simulink model "Mobile_robot_2wheels_PID_4_10_V0_2018 (1)"  (R2018b)
settings: Solver=VariableStepAuto  StartTime=0.0  StopTime=25  FixedStep=0.0001  MaxStep=0.01  RelTol=1e-3
libraries: fuzblock x6, simulink x4
settings Model: Creator=HP-PC  LastModifiedBy=thetr
settings DebuggingCC: SFMachineParentedDataDiag=error

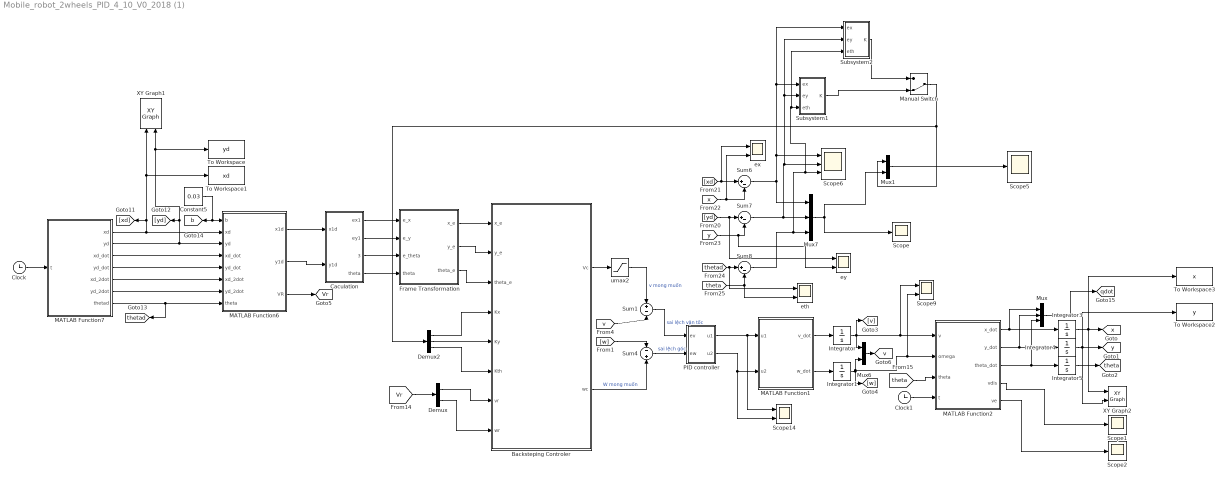
== system Mobile_robot_2wheels_PID_4_10_V0_2018 (1) ==
  Backsteping Controler : MATLAB Function  TreatAsAtomicUnit=on
  Caculation : Subsystem
  Clock : Clock
  Clock1 : Clock
  Constant5 : Constant  Value=0.03
  Demux : Demux  Outputs=2
  Demux2 : Demux  Outputs=3
  Frame Transformation : MATLAB Function  TreatAsAtomicUnit=on
  Integrator{,1,3..5} (5 alike) : Integrator
  MATLAB Function1 : MATLAB Function  TreatAsAtomicUnit=on
  MATLAB Function2 : MATLAB Function  TreatAsAtomicUnit=on
  MATLAB Function6 : MATLAB Function  TreatAsAtomicUnit=on
  MATLAB Function7 : MATLAB Function  TreatAsAtomicUnit=on
  Manual Switch : ManualSwitch  CurrentSetting=0
  Mux : Mux  Inputs=3
  Mux1 : Mux  Inputs=2
  Mux6 : Mux  Inputs=2
  Mux7 : Mux  Inputs=3
  PID controller : Subsystem
  Scope{,1..2,5} (4 alike) : Scope
  Scope14 : Scope  NumInputPorts=2
  Scope6 : Scope  NumInputPorts=3
  Scope9 : Scope  NumInputPorts=2
  Subsystem1 : Subsystem
  Subsystem2 : Subsystem
  Sum1 : Sum  Inputs=+-
  Sum4 : Sum  Inputs=-+
  Sum6 : Sum  Inputs=|+-
  Sum7 : Sum  Inputs=|+-
  Sum8 : Sum  Inputs=|+-
  To Workspace : ToWorkspace  VariableName=yd  SampleTime=-1
  To Workspace1 : ToWorkspace  VariableName=xd  SampleTime=-1
  To Workspace2 : ToWorkspace  VariableName=y  SampleTime=-1
  To Workspace3 : ToWorkspace  VariableName=x  SampleTime=-1
  XY Graph1 : simulink/Sinks/XY Graph  xmin=-20  xmax=20  ymin=-20  ymax=20  st=-1
  XY Graph2 : simulink/Sinks/XY Graph  xmin=-20  xmax=20  ymin=-20  ymax=20  st=-1
  eth : Scope  NumInputPorts=2
  ex : Scope  NumInputPorts=2
  ey : Scope  NumInputPorts=2
  umax2 : Saturate  UpperLimit=3  LowerLimit=-3
  tag scope: Vr=global, b=global, qdot=global, theta=global, thetad=global, v=global, x=global, y=global
  wires:
  Integrator4/1 -> To Workspace2/1, XY Graph2/2, [y]
  Integrator5/1 -> [theta]
  Integrator3/1 -> To Workspace3/1, XY Graph2/1, [x]
  MATLAB Function7/1(xd) -> To Workspace1/1, XY Graph1/1, [xd], MATLAB Function6/2(xd)
  MATLAB Function2/3(theta_dot) -> Mux/3, Integrator5/1
  MATLAB Function2/1(x_dot) -> Integrator3/1, Mux/1
  PID controller/2(u2) -> Scope14/2, MATLAB Function1/2(u2)
  Demux2/2 -> Backsteping Controler/5(Ky)
  Frame Transformation/3(theta_e) -> Backsteping Controler/3(theta_e)
  PID controller/1(u1) -> Scope14/1, MATLAB Function1/1(u1)
  MATLAB Function1/2(w_dot) -> Integrator1/1
  Clock/1 -> MATLAB Function7/1(t)
  Constant5/1 -> MATLAB Function6/1(b), [b]
  MATLAB Function7/3(xd_dot) -> MATLAB Function6/4(xd_dot)
  MATLAB Function7/7(thetad) -> [thetad], MATLAB Function6/8(theta)
  Mux7/1 -> Scope/1, Mux1/2
  Sum1/1 -> PID controller/1(ev)  "sai lệch vận tốc"
  [x] -> ex/2, Sum6/2
  MATLAB Function7/2(yd) -> To Workspace/1, XY Graph1/2, [yd], MATLAB Function6/3(yd)
  Sum8/1 -> Subsystem2/3(eth), Subsystem1/3(eth), Scope6/3, Mux7/3
  [Vr] -> Demux/1
  [thetad] -> eth/1, Sum8/1
  Integrator1/1 -> Mux6/2, Scope9/2, MATLAB Function2/2(omega), [w]
  [xd] -> ex/1, Sum6/1
  Sum4/1 -> PID controller/2(ew)  "sai lệch góc"
  Frame Transformation/2(y_e) -> Backsteping Controler/2(y_e)
  Demux2/1 -> Backsteping Controler/4(Kx)
  [v] -> Sum1/2
  Caculation/4(theta) -> Frame Transformation/4(theta)
  Demux/2 -> Backsteping Controler/8(wr)
  [w] -> Sum4/1
  MATLAB Function1/1(v_dot) -> Integrator/1
  MATLAB Function6/1(x1d) -> Caculation/1(x1d)
  Caculation/1(ex1) -> Frame Transformation/1(e_x)
  MATLAB Function7/4(yd_dot) -> MATLAB Function6/5(yd_dot)
  Demux2/3 -> Backsteping Controler/6(Kth)
  Mux/1 -> [qdot]
  Demux/1 -> Backsteping Controler/7(vr)
  MATLAB Function6/3(VR) -> [Vr]
  [theta] -> eth/2, Sum8/2
  Clock1/1 -> MATLAB Function2/4(t)
  Frame Transformation/1(x_e) -> Backsteping Controler/1(x_e)
  umax2/1 -> Sum1/1  "v mong muốn"
  Integrator/1 -> [v], Scope9/1, MATLAB Function2/1(v), Mux6/1
  MATLAB Function7/5(xd_2dot) -> MATLAB Function6/6(xd_2dot)
  MATLAB Function7/6(yd_2dot) -> MATLAB Function6/7(yd_2dot)
  [theta] -> MATLAB Function2/3(theta)
  Caculation/3(etheta1) -> Frame Transformation/3(e_theta)
  MATLAB Function6/2(y1d) -> Caculation/2(y1d)
  MATLAB Function2/2(y_dot) -> Mux/2, Integrator4/1
  Caculation/2(ey1) -> Frame Transformation/2(e_y)
  Sum6/1 -> Subsystem2/1(ex), Subsystem1/1(ex), Scope6/1, Mux7/1
  Mux6/1 -> [v]
  [yd] -> ey/1, Sum7/1
  Backsteping Controler/1(Vc) -> umax2/1
  Sum7/1 -> Scope6/2, Subsystem2/2(ey), Subsystem1/2(ey), Mux7/2
  Backsteping Controler/2(wc) -> Sum4/2  "W mong muốn"
  Subsystem1/1(K) -> Manual Switch/2
  Mux1/1 -> Scope5/1
  MATLAB Function2/4(vdis) -> Scope1/1
  MATLAB Function2/5(ve) -> Scope2/1
  [y] -> ey/2, Sum7/2
  Subsystem2/1(K) -> Manual Switch/1
  Manual Switch/1 -> Demux2/1, Mux1/1

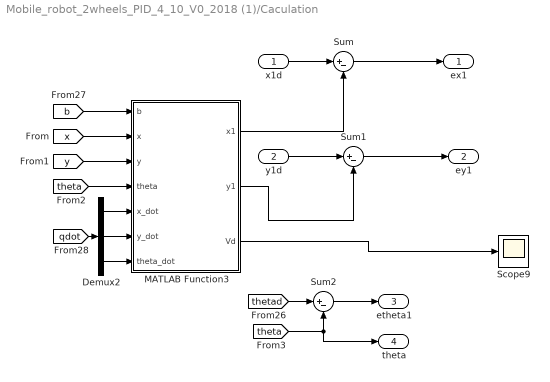
== system Mobile_robot_2wheels_PID_4_10_V0_2018 (1)/Caculation ==
  x1d : Inport
  y1d : Inport  Port=2
  Demux2 : Demux  Outputs=3
  MATLAB Function3 : MATLAB Function  TreatAsAtomicUnit=on
  Scope9 : Scope
  Sum : Sum  Inputs=|+-
  Sum1 : Sum  Inputs=|+-
  Sum2 : Sum  Inputs=|+-
  ex1 : Outport  VectorParamsAs1DForOutWhenUnconnected=on
  ey1 : Outport  Port=2  VectorParamsAs1DForOutWhenUnconnected=on
  etheta1 : Outport  Port=3  VectorParamsAs1DForOutWhenUnconnected=on
  theta : Outport  Port=4  VectorParamsAs1DForOutWhenUnconnected=on
  wires:
  Demux2/3 -> MATLAB Function3/7(theta_dot)
  MATLAB Function3/3(Vd) -> Scope9/1
  [y] -> MATLAB Function3/3(y)
  Sum/1 -> ex1/1
  MATLAB Function3/2(y1) -> Sum1/2
  MATLAB Function3/1(x1) -> Sum/2
  [x] -> MATLAB Function3/2(x)
  Demux2/2 -> MATLAB Function3/6(y_dot)
  [theta] -> MATLAB Function3/4(theta)
  [b] -> MATLAB Function3/1(b)
  Demux2/1 -> MATLAB Function3/5(x_dot)
  [qdot] -> Demux2/1
  Sum1/1 -> ey1/1
  y1d/1 -> Sum1/1
  x1d/1 -> Sum/1
  [thetad] -> Sum2/1
  [theta] -> theta/1, Sum2/2
  Sum2/1 -> etheta1/1

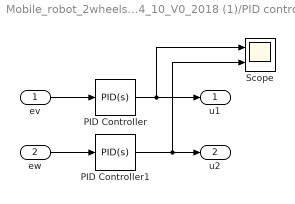
== system Mobile_robot_2wheels_PID_4_10_V0_2018 (1)/PID controller ==
  ev : Inport
  ew : Inport  Port=2
  PID Controller : simulink/Continuous/PID Controller  Controller=PID  Form=Parallel  TimeDomain=Continuous-time  SampleTime=-1  IntegratorMethod=Forward Euler  FilterMethod=Forward Euler  ControllerParametersSource=internal  P=100  I=10  D=0.1  UseFilter=on  N=193.352804132204  TunerSelectOption=Transfer Function Based (PID Tuner App)  InitialConditionSource=internal  InitialConditionForIntegrator=0  InitialConditionForFilter=0  DifferentiatorICPrevScaledInput=0  ExternalReset=none  TrackingMode=off  Kt=1  LimitOutput=off  UpperSaturationLimit=inf  LowerSaturationLimit=-inf  LinearizeAsGain=on  AntiWindupMode=none  Kb=1  POutMin=[]  POutMax=[]  IOutMin=[]  IOutMax=[]  DOutMin=[]  DOutMax=[]  NOutMin=[]  NOutMax=[]  SumOutMin=[]  SumOutMax=[]  SaturationOutMin=[]  SaturationOutMax=[]  PParamMin=[]  PParamMax=[]  IParamMin=[]  IParamMax=[]  DParamMin=[]  DParamMax=[]  NParamMin=[]  NParamMax=[]  KbParamMin=[]  KbParamMax=[]  KtParamMin=[]  KtParamMax=[]  KbOutMin=[]  KbOutMax=[]  KtOutMin=[]  KtOutMax=[]  IntegratorOutMin=[]  IntegratorOutMax=[]  FilterOutMin=[]  FilterOutMax=[]  SumI1OutMin=[]  SumI1OutMax=[]  SumI2OutMin=[]  SumI2OutMax=[]  SumI3OutMin=[]  SumI3OutMax=[]  SumI4OutMin=[]  SumI4OutMax=[]  SumDOutMin=[]  SumDOutMax=[]  DifferentiatorOutMin=[]  DifferentiatorOutMax=[]  FilterDiffOutCoefMin=[]  FilterDiffOutCoefMax=[]  ReciprocalOutMin=[]  ReciprocalOutMax=[]  SumDenOutMin=[]  SumDenOutMax=[]  SumNumOutMin=[]  SumNumOutMax=[]  DivideOutMin=[]  DivideOutMax=[]  IntegratorContinuousStateAttributes=''  IntegratorStateMustResolveToSignalObject=off  IntegratorRTWStateStorageClass=Auto  FilterContinuousStateAttributes=''  FilterStateMustResolveToSignalObject=off  FilterRTWStateStorageClass=Auto  ParallelPVariant=InternalParameters  IdealPVariant=Disabled  IVariant=InternalParameters  DVariant=InternalParameters  IntegratorVariant=Continuous  SatVariant=Disabled  AWVariant=Passthrough  PCopyVariant=Disabled  TRVariant=Disabled  FdbkBlocksVariant=Forward  IdealPFdbkVariant=Disabled  SatFdbkVariant=Disabled  DerivativeFilterVariant=ContFilter  NVariant=InternalParameters  NCopyVariant=Disabled  FilterICVariant=InternalICsFilter  IntegratorICVariant=InternalICs  ExternalResetVariant=Disabled  TRSumVariant=Passthrough  SumFdbkVariant=Disabled  SumVariant=Sum_PID
  PID Controller1 : simulink/Continuous/PID Controller  Controller=PID  Form=Parallel  TimeDomain=Continuous-time  SampleTime=-1  IntegratorMethod=Forward Euler  FilterMethod=Forward Euler  ControllerParametersSource=internal  P=100  I=10  D=0.1  UseFilter=on  N=3867.05608255163  TunerSelectOption=Transfer Function Based (PID Tuner App)  InitialConditionSource=internal  InitialConditionForIntegrator=0  InitialConditionForFilter=0  DifferentiatorICPrevScaledInput=0  ExternalReset=none  TrackingMode=off  Kt=1  LimitOutput=off  UpperSaturationLimit=inf  LowerSaturationLimit=-inf  LinearizeAsGain=on  AntiWindupMode=none  Kb=1  POutMin=[]  POutMax=[]  IOutMin=[]  IOutMax=[]  DOutMin=[]  DOutMax=[]  NOutMin=[]  NOutMax=[]  SumOutMin=[]  SumOutMax=[]  SaturationOutMin=[]  SaturationOutMax=[]  PParamMin=[]  PParamMax=[]  IParamMin=[]  IParamMax=[]  DParamMin=[]  DParamMax=[]  NParamMin=[]  NParamMax=[]  KbParamMin=[]  KbParamMax=[]  KtParamMin=[]  KtParamMax=[]  KbOutMin=[]  KbOutMax=[]  KtOutMin=[]  KtOutMax=[]  IntegratorOutMin=[]  IntegratorOutMax=[]  FilterOutMin=[]  FilterOutMax=[]  SumI1OutMin=[]  SumI1OutMax=[]  SumI2OutMin=[]  SumI2OutMax=[]  SumI3OutMin=[]  SumI3OutMax=[]  SumI4OutMin=[]  SumI4OutMax=[]  SumDOutMin=[]  SumDOutMax=[]  DifferentiatorOutMin=[]  DifferentiatorOutMax=[]  FilterDiffOutCoefMin=[]  FilterDiffOutCoefMax=[]  ReciprocalOutMin=[]  ReciprocalOutMax=[]  SumDenOutMin=[]  SumDenOutMax=[]  SumNumOutMin=[]  SumNumOutMax=[]  DivideOutMin=[]  DivideOutMax=[]  IntegratorContinuousStateAttributes=''  IntegratorStateMustResolveToSignalObject=off  IntegratorRTWStateStorageClass=Auto  FilterContinuousStateAttributes=''  FilterStateMustResolveToSignalObject=off  FilterRTWStateStorageClass=Auto  ParallelPVariant=InternalParameters  IdealPVariant=Disabled  IVariant=InternalParameters  DVariant=InternalParameters  IntegratorVariant=Continuous  SatVariant=Disabled  AWVariant=Passthrough  PCopyVariant=Disabled  TRVariant=Disabled  FdbkBlocksVariant=Forward  IdealPFdbkVariant=Disabled  SatFdbkVariant=Disabled  DerivativeFilterVariant=ContFilter  NVariant=InternalParameters  NCopyVariant=Disabled  FilterICVariant=InternalICsFilter  IntegratorICVariant=InternalICs  ExternalResetVariant=Disabled  TRSumVariant=Passthrough  SumFdbkVariant=Disabled  SumVariant=Sum_PID
  Scope : Scope  NumInputPorts=2
  u1 : Outport
  u2 : Outport  Port=2
  wires:
  ev/1 -> PID Controller/1
  ew/1 -> PID Controller1/1
  PID Controller/1 -> Scope/1, u1/1
  PID Controller1/1 -> Scope/2, u2/1

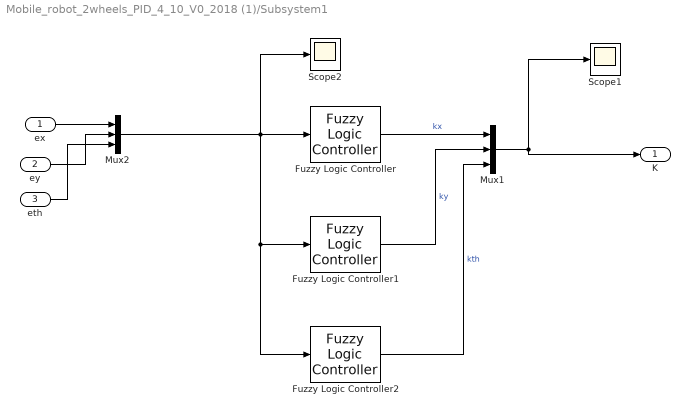
== system Mobile_robot_2wheels_PID_4_10_V0_2018 (1)/Subsystem1 ==
  ex : Inport
  ey : Inport  Port=2
  eth : Inport  Port=3
  Fuzzy Logic Controller : fuzblock/Fuzzy Logic  Controller  FIS='FUZZY1_1.fis'  OutputSampleNumber=101  DataType=double  FuzzifiedInputs=off  RuleFiringStrengths=off  RuleOutputs=off  AggregatedOutputs=off  SimulateUsing=Interpreted execution  OutOfRangeInputValueMessage=warning  NoRuleFiredMessage=warning  EmptyOutputFuzzySetMessage=warning
  Fuzzy Logic Controller1 : fuzblock/Fuzzy Logic  Controller  FIS='FUZZY1_2.fis'  OutputSampleNumber=101  DataType=double  FuzzifiedInputs=off  RuleFiringStrengths=off  RuleOutputs=off  AggregatedOutputs=off  SimulateUsing=Interpreted execution  OutOfRangeInputValueMessage=warning  NoRuleFiredMessage=warning  EmptyOutputFuzzySetMessage=warning
  Fuzzy Logic Controller2 : fuzblock/Fuzzy Logic  Controller  FIS='FUZZY1_3.fis'  OutputSampleNumber=101  DataType=double  FuzzifiedInputs=off  RuleFiringStrengths=off  RuleOutputs=off  AggregatedOutputs=off  SimulateUsing=Interpreted execution  OutOfRangeInputValueMessage=warning  NoRuleFiredMessage=warning  EmptyOutputFuzzySetMessage=warning
  Mux1 : Mux  Inputs=3
  Mux2 : Mux  Inputs=3
  Scope1 : Scope
  Scope2 : Scope
  K : Outport  VectorParamsAs1DForOutWhenUnconnected=on
  wires:
  Fuzzy Logic Controller/1 -> Mux1/1  "kx"
  Fuzzy Logic Controller2/1 -> Mux1/3  "kth"
  Fuzzy Logic Controller1/1 -> Mux1/2  "ky"
  Mux1/1 -> K/1, Scope1/1
  ex/1 -> Mux2/1
  Mux2/1 -> Fuzzy Logic Controller2/1, Fuzzy Logic Controller1/1, Scope2/1, Fuzzy Logic Controller/1
  ey/1 -> Mux2/2
  eth/1 -> Mux2/3

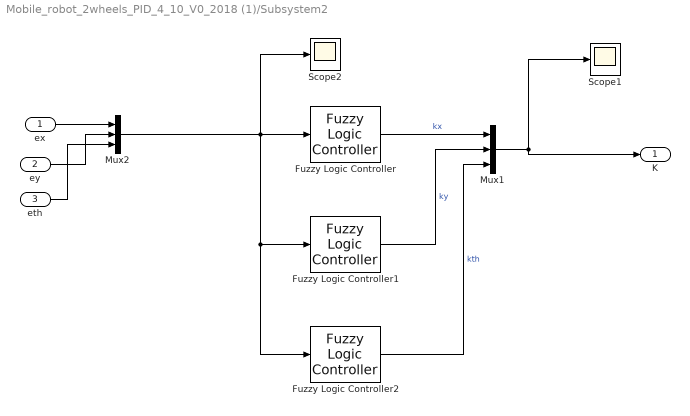
== system Mobile_robot_2wheels_PID_4_10_V0_2018 (1)/Subsystem2 ==
  ex : Inport
  ey : Inport  Port=2
  eth : Inport  Port=3
  Fuzzy Logic Controller : fuzblock/Fuzzy Logic  Controller  FIS='LUAT9B1.fis'  OutputSampleNumber=101  DataType=double  FuzzifiedInputs=off  RuleFiringStrengths=off  RuleOutputs=off  AggregatedOutputs=off  SimulateUsing=Interpreted execution  OutOfRangeInputValueMessage=warning  NoRuleFiredMessage=warning  EmptyOutputFuzzySetMessage=warning
  Fuzzy Logic Controller1 : fuzblock/Fuzzy Logic  Controller  FIS='LUAT9B2.fis'  OutputSampleNumber=101  DataType=double  FuzzifiedInputs=off  RuleFiringStrengths=off  RuleOutputs=off  AggregatedOutputs=off  SimulateUsing=Interpreted execution  OutOfRangeInputValueMessage=warning  NoRuleFiredMessage=warning  EmptyOutputFuzzySetMessage=warning
  Fuzzy Logic Controller2 : fuzblock/Fuzzy Logic  Controller  FIS='LUAT9B3.fis'  OutputSampleNumber=101  DataType=double  FuzzifiedInputs=off  RuleFiringStrengths=off  RuleOutputs=off  AggregatedOutputs=off  SimulateUsing=Interpreted execution  OutOfRangeInputValueMessage=warning  NoRuleFiredMessage=warning  EmptyOutputFuzzySetMessage=warning
  Mux1 : Mux  Inputs=3
  Mux2 : Mux  Inputs=3
  Scope1 : Scope
  Scope2 : Scope
  K : Outport  VectorParamsAs1DForOutWhenUnconnected=on
  wires:
  eth/1 -> Mux2/3
  ey/1 -> Mux2/2
  Mux2/1 -> Fuzzy Logic Controller/1, Scope2/1, Fuzzy Logic Controller1/1, Fuzzy Logic Controller2/1
  ex/1 -> Mux2/1
  Mux1/1 -> Scope1/1, K/1
  Fuzzy Logic Controller1/1 -> Mux1/2  "ky"
  Fuzzy Logic Controller2/1 -> Mux1/3  "kth"
  Fuzzy Logic Controller/1 -> Mux1/1  "kx"

== matlab function Mobile_robot_2wheels_PID_4_10_V0_2018 (1)/Frame Transformation ==
  data: e_x input; x_e output; e_y input; e_theta input; y_e output; theta_e output; theta input
function [x_e,y_e,theta_e] = fcn(e_x,e_y,e_theta,theta)
A=[cos(theta) sin(theta) 0;-sin(theta) cos(theta) 0;0 0 1];
B=[e_x;e_y;e_theta];
C=A*B;
x_e=C(1);
y_e=C(2);
theta_e=C(3);
% công thức 45

== matlab function Mobile_robot_2wheels_PID_4_10_V0_2018 (1)/Backsteping Controler ==
  data: x_e input; Vc output; y_e input; theta_e input; Kx input; Ky input; Kth input; wc output; vr input; wr input
function [Vc,wc] = fcn(x_e,y_e,theta_e,Kx,Ky,Kth,vr,wr)
Vc=vr*cos(theta_e)+ Kx*x_e;
wc=wr+vr*Ky*y_e + Kth*sin(theta_e);
% công thức 46

== matlab function Mobile_robot_2wheels_PID_4_10_V0_2018 (1)/Caculation/MATLAB Function3 ==
  data: b input; x1 output; y1 output; x input; y input; theta input; x_dot input; y_dot input; theta_dot input; Vd output
function [x1,y1,Vd] = q1(b,x,y,theta,x_dot,y_dot,theta_dot)
%% Thiet lap quy dao chuyen dong cho robot
%theta=atan2(yd_dot,xd_dot);
x1=x+b*cos(theta);
y1=y+b*sin(theta);

x1_dot=x_dot-b*theta_dot*sin(theta);
y1_dot=y_dot+b*theta_dot*cos(theta);

Td=[cos(theta) -b*sin(theta); sin(theta) b*cos(theta)];
Vd=Td\[x1_dot; y1_dot];

== matlab function Mobile_robot_2wheels_PID_4_10_V0_2018 (1)/MATLAB Function1 ==
  data: u1 input; v_dot output; u2 input; w_dot output
function [v_dot,w_dot]=fcn(u1,u2)
m=15;I=2.5;r=0.1; R=0.5;
M=[m 0;0 I];
T=[1/(r*m) 0;0 R/(r*I)];
u=[u1;u2];
N=T*u;
Z=M\N;
v_dot=Z(1);
w_dot=Z(2);

== matlab function Mobile_robot_2wheels_PID_4_10_V0_2018 (1)/MATLAB Function2 ==
  data: v input; x_dot output; omega input; theta input; y_dot output; theta_dot output; vdis output; ve output; t input
function [x_dot,y_dot,theta_dot,vdis,ve]=Kinematics(v,omega,theta,t)
S=[cos(theta) 0;sin(theta) 0;0 1];
ve0=[v;omega];
if t>10%&&t<50
    vdis0=[0*v;0*omega];
else
    vdis0=[0;0];  
end
ve=ve0-vdis0;
vdis=vdis0;
qdot=S*ve;

x_dot=qdot(1);
y_dot=qdot(2);
theta_dot=qdot(3);

== matlab function Mobile_robot_2wheels_PID_4_10_V0_2018 (1)/MATLAB Function6 ==
  data: b input; x1d output; y1d output; xd input; yd input; xd_dot input; yd_dot input; xd_2dot input; yd_2dot input; theta input; VR output
function [x1d,y1d,VR] = quydao(b,xd,yd,xd_dot,yd_dot,xd_2dot,yd_2dot,theta)
%% Thiet lap quy dao chuyen dong cho robot
%theta=atan2(yd_dot,xd_dot);
x1d=xd+b*cos(theta);
y1d=yd+b*sin(theta);
wd=(yd_2dot*xd_dot - xd_2dot*yd_dot)/(xd_dot^2+yd_dot^2);
x1d_dot=xd_dot-b*wd*sin(theta);
y1d_dot=yd_dot+b*wd*cos(theta);
thetad_dot=wd;
Td=[cos(theta) -b*sin(theta); sin(theta) b*cos(theta)];
VR=Td\[x1d_dot; y1d_dot];

== matlab function Mobile_robot_2wheels_PID_4_10_V0_2018 (1)/MATLAB Function7 ==
  data: t input; xd output; yd output; xd_dot output; yd_dot output; xd_2dot output; yd_2dot output; thetad output
function [xd,yd,xd_dot,yd_dot,xd_2dot,yd_2dot,thetad] = quydao(t)
%% Khoi tao quy dao chuyen dong
R=5; %ban kinh quy dao
w=0.3; %rad/s =2*pi*f f=w/2/pi -> T=1/f
xd=R*cos(w*t);
yd=R*sin(w*t);
xd_dot=-R*w*sin(w*t);
yd_dot=R*w*cos(w*t);
x0d_dot=-R*w*sin(w);
y0d_dot=R*w*cos(w);
xd_2dot=-R*w^2*cos(w*t);
yd_2dot=-R*w^2*sin(w*t);
theta0=atan2(y0d_dot,x0d_dot)-w;
thetad=w*t + theta0;
